simulink model "semnal"  (R2018b)
settings: Solver=FixedStepDiscrete  StartTime=0.0  StopTime=10.0  FixedStep=0.01  RelTol=1e-3
libraries: simulink x2
settings Model: Creator=Adrian  LastModifiedBy=ganea

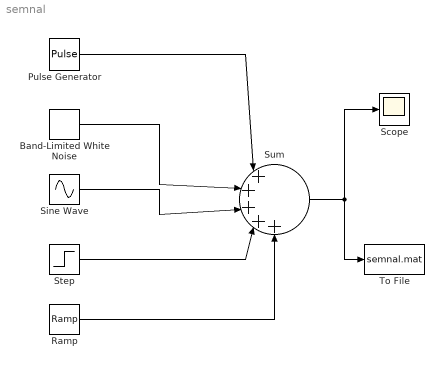
== system semnal ==
  Band-Limited White Noise : simulink/Sources/Band-Limited White Noise  Cov=[0.0002]  Ts=0.01  seed=[23341]
  Pulse Generator : DiscretePulseGenerator  PulseType=Time based  Amplitude=5  Period=4  PulseWidth=0.5  PhaseDelay=2
  Ramp : simulink/Sources/Ramp  slope=0.2  start=5  InitialOutput=0
  Scope : Scope
  Sine Wave : Sin  SampleTime=0
  Step : Step  Time=3  After=3  SampleTime=0
  Sum : Sum  Inputs=|+++++
  To File : ToFile  Filename=semnal.mat  MatrixName=y
  wires:
  Pulse Generator/1 -> Sum/1
  Band-Limited White Noise/1 -> Sum/2
  Sine Wave/1 -> Sum/3
  Step/1 -> Sum/4
  Ramp/1 -> Sum/5
  Sum/1 -> To File/1, Scope/1
